simulink model "User_Input"  (R2015a)
settings: Solver=FixedStepDiscrete  SolverMode=SingleTasking  StartTime=0.0  StopTime=inf  FixedStep=0.004  MaxStep=0.004  RelTol=1e-3
settings Model: CovSFcnEnable=off  Creator=ADAM  LastModifiedBy=denise
settings SolverCC: ExtrapolationOrder=1
settings DataIOCC: LimitDataPoints=off  MaxDataPoints=1  SaveFormat=Structure  SignalLoggingSaveFormat=ModelDataLogs  SaveOutput=off  DSMLogging=off  SaveTime=off  OutputSaveName=model_out  SignalLoggingName=model_out
settings OptimizationCC: ExpressionDepthLimit=2147483647  SimCompilerOptimization=on
settings DebuggingCC: UnderspecifiedInitializationDetection=Classic  MergeDetectMultiDrivingBlocksExec=none  SolverPrmCheckMsg=warning  InheritedTsInSrcMsg=none  MultiTaskDSMMsg=warning  MultiTaskCondExecSysMsg=none  UnconnectedInputMsg=none  UnconnectedOutputMsg=none  UnconnectedLineMsg=none  StateNameClashWarn=warning
settings HardwareCC: ProdIntDivRoundTo=Zero  ProdEndianess=LittleEndian  ProdHWDeviceType=Generic->32-bit x86 compatible
settings CodeAppCC: MaxIdLength=95
settings GRTTargetCC: MatFileLogging=off

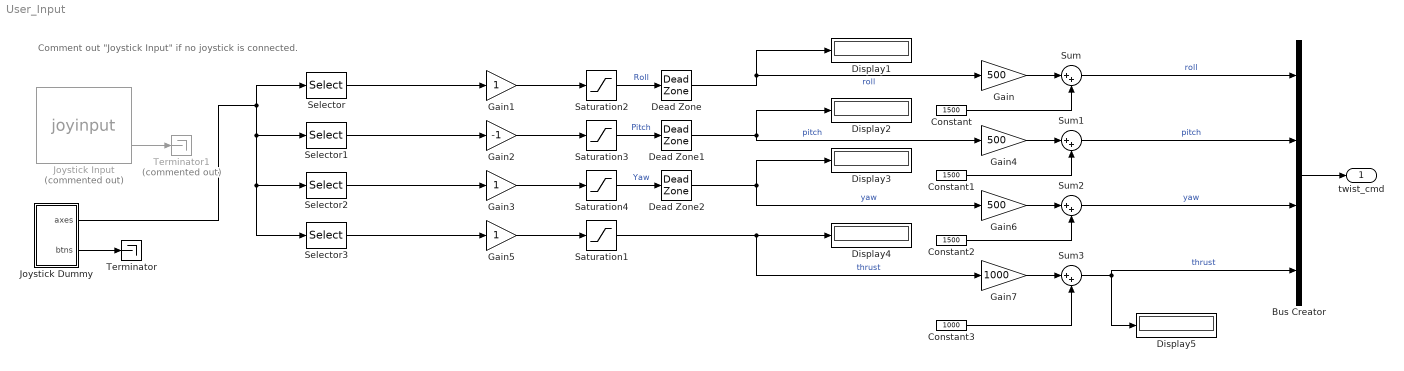
== system User_Input ==
  note: Comment out "Joystick Input" if no joystick is connected.
  Bus Creator : BusCreator  OutDataTypeStr=Bus: Twist_Bus
  Constant : Constant  Value=1500
  Constant1 : Constant  Value=1500
  Constant2 : Constant  Value=1500
  Constant3 : Constant  Value=1000
  Dead Zone : DeadZone  LowerValue=-0.1  UpperValue=0.1  SaturateOnIntegerOverflow=on
  Dead Zone1 : DeadZone  LowerValue=-0.1  UpperValue=0.1  SaturateOnIntegerOverflow=on
  Dead Zone2 : DeadZone  LowerValue=-0.1  UpperValue=0.1  SaturateOnIntegerOverflow=on
  Display{1..5} (5 alike) : Display
  Gain : Gain  Gain=500
  Gain1 : Gain  OutDataTypeStr=double
  Gain2 : Gain  Gain=-1  OutDataTypeStr=double
  Gain3 : Gain  OutDataTypeStr=double
  Gain4 : Gain  Gain=500
  Gain5 : Gain  OutDataTypeStr=double
  Gain6 : Gain  Gain=500
  Gain7 : Gain  Gain=1000
  Joystick Dummy : Subsystem
  Joystick Input : S-Function  Commented=on  FunctionName=joyinput  Parameters=joyid, adjustports, forcefeed  mask(Joystick Input){joyid=1, adjustports=on, forcefeed=off}
      mask prompts: joyid "Joystick ID:"; adjustports "Adjust I/O ports according to joystick capabilities"; forcefeed "Enable force-feedback input"
      mask help: Joystick input device driver.
      mask init:
      | label = 'image(imread(''joystickicon.png'')); port_label(''output'', 1, ''Axes''); port_label(''output'', 2, ''Buttons''); ';
      | porthandles = get_param(gcbh, 'PortHandles');
      | if numel(porthandles.Outport)>2
      |   label = [label 'port_label(''output'', 3, ''Point of View''); '];
      | end
      | if numel(porthandles.Inport)>0  label = [label 'port_label(''input'', 1, ''Force''); '];
      | end
      | set_param(gcbh, 'MaskDisplay', label);
      settings: CopyFcn=if ~vrmfunc('islibrary',gcbh) set_param(gcbh,'adjustports','on'); end
      mask Help: helpview(vrmfunc('FnHelpTopic'), 'vr_joystickinput');
      mask Display: image(imread('joystickicon.png')); port_label('output', 1, 'Axes'); port_label('output', 2, 'Buttons');
  Saturation{1..4} (4 alike) : Saturate  UpperLimit=1  LowerLimit=-1
  Selector : Selector  Indices=[4]
  Selector1 : Selector  Indices=[5]
  Selector2 : Selector  Indices=[1]
  Selector3 : Selector  Indices=[3]
  Sum{,1..3} (4 alike) : Sum  Inputs=|++
  Terminator : Terminator
  Terminator1 : Terminator  Commented=on
  twist_cmd : Outport  OutDataTypeStr=Bus: Twist_Bus
  wires:
  Joystick Dummy/2(btns) -> Terminator/1
  Sum2/1 -> Bus Creator/3  "yaw"
  Gain7/1 -> Sum3/1
  Sum1/1 -> Bus Creator/2  "pitch"
  Constant1/1 -> Sum1/2
  Gain6/1 -> Sum2/1
  Sum3/1 -> Bus Creator/4, Display5/1  "thrust"
  Constant2/1 -> Sum2/2
  Joystick Input/2 -> Terminator1/1
  Saturation4/1 -> Dead Zone2/1  "Yaw"
  Joystick Dummy/1(axes) -> Selector3/1, Selector2/1, Selector1/1, Selector/1
  Constant3/1 -> Sum3/2
  Gain2/1 -> Saturation3/1
  Selector1/1 -> Gain2/1
  Gain5/1 -> Saturation1/1
  Dead Zone1/1 -> Display2/1, Gain4/1  "pitch"
  Dead Zone2/1 -> Display3/1, Gain6/1  "yaw"
  Saturation1/1 -> Display4/1, Gain7/1  "thrust"
  Selector3/1 -> Gain5/1
  Constant/1 -> Sum/2
  Selector/1 -> Gain1/1
  Gain/1 -> Sum/1
  Gain4/1 -> Sum1/1
  Selector2/1 -> Gain3/1
  Saturation3/1 -> Dead Zone1/1  "Pitch"
  Dead Zone/1 -> Display1/1, Gain/1  "roll"
  Saturation2/1 -> Dead Zone/1  "Roll"
  Gain3/1 -> Saturation4/1
  Gain1/1 -> Saturation2/1
  Sum/1 -> Bus Creator/1  "roll"
  Bus Creator/1 -> twist_cmd/1

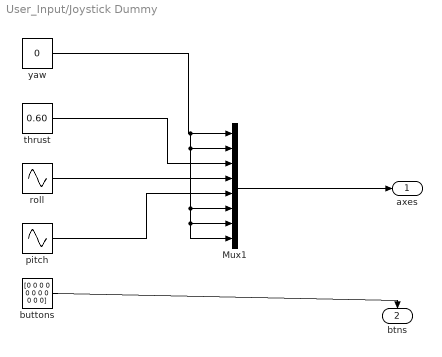
== system User_Input/Joystick Dummy ==
  Mux1 : Mux  Inputs=8
  buttons : Constant  Value=[0 0 0 0 0 0 0 0 0 0 0]
  pitch : Sin  Amplitude=0.605  Frequency=0.5  Phase=pi  SampleTime=0.004
  roll : Sin  Amplitude=0.28  Frequency=0.5  Phase=1.57  SampleTime=0.004
  thrust : Constant  Value=0.60
  yaw : Constant  Value=0
  axes : Outport
  btns : Outport  Port=2
  wires:
  buttons/1 -> btns/1
  Mux1/1 -> axes/1
  roll/1 -> Mux1/4
  thrust/1 -> Mux1/3
  pitch/1 -> Mux1/5
  yaw/1 -> Mux1/1, Mux1/2, Mux1/6, Mux1/7, Mux1/8
